simulink model "Simulink_Simulation"  (Simulink 10.1)
settings: Solver=ode23tb  StartTime=0.0  StopTime=3  RelTol=1e-3  EnableMultiTasking=on
undefined symbols (not defined in the file or in its folder): sigbuilder_block
libraries: powerlib x10, powerlib_meascontrol x1
settings Model: Creator=asus1  LastModifiedBy=x64
settings DataIOCC: LimitDataPoints=on
settings DebuggingCC: UnderspecifiedInitializationDetection=Simplified  MergeDetectMultiDrivingBlocksExec=error  SolverPrmCheckMsg=warning
settings GRTTargetCC: CombineOutputUpdateFcns=on  GRTInterface=off
settings ConfigComp: CovSFcnEnable=off
settings SimscapeCC: SimscapeNormalizeSystem=off

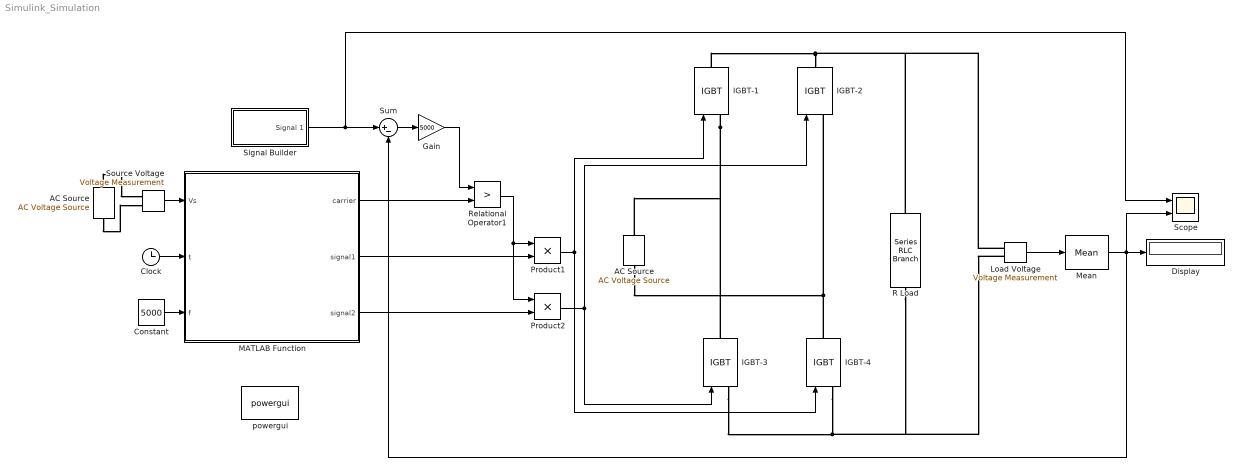
== system Simulink_Simulation ==
  AC Source : powerlib/Electrical Sources/AC Voltage Source  Amplitude=220*sqrt(2)  Phase=0  Frequency=50  SampleTime=0  Measurements=None  BusType=swing  Pref=10e3  Qref=0  Qmin=-inf  Qmax=+inf
  "AC Source " : powerlib/Electrical Sources/AC Voltage Source  Amplitude=220*sqrt(2)  Phase=0  Frequency=50  SampleTime=0  Measurements=None  BusType=swing  Pref=10e3  Qref=0  Qmin=-inf  Qmax=+inf
  "Clock " : Clock
  "Constant " : Constant  Value=5000
  "Display " : Display
  Gain : Gain  Gain=5000
  IGBT-{1..4} (4 alike) : powerlib/Power Electronics/IGBT  Ron=0.001  Lon=0  Vf=0.001  Tf=1e-6  Tt=2e-6  IC=0  Rs=1e5  Cs=inf  Measurements=off
  Load Voltage : powerlib/Measurements/Voltage Measurement  PhasorSimulation=off  OutputType=Complex  PSBequivalent=0
  "MATLAB Function " : MATLAB Function  TreatAsAtomicUnit=on
  Mean : powerlib_meascontrol/Measurements/Mean  Freq=50  Vinit=0  Ts=0
  Product1 : Product
  Product2 : Product
  R Load : powerlib/Elements/Series RLC Branch  LConnTagsString=__new0  RConnTagsString=__new0  BranchType=R  Resistance=10  Inductance=1e-3  SetiL0=off  InitialCurrent=0  Capacitance=1e-6  Setx0=off  InitialVoltage=0  Measurements=None
  Relational Operator1 : RelationalOperator  Operator=>  OutDataTypeStr=boolean  RndMeth=Nearest
  "Scope " : Scope  NumInputPorts=2
  "Signal Builder " : Subsystem  Tag=STV Subsys  LoadFcn=sigbuilder_block('load');  StartFcn=sigbuilder_block('start');  StopFcn=sigbuilder_block('stop');  ClipboardFcn=sigbuilder_block('clipboard');  mask(Sigbuilder block){tuvar=[0:10]}
      mask help: Simulink:masks:SigbuilderBlock_MD
      mask init:
      | if ~strcmp(get_param(bdroot(gcbh),'SimulationStatus'),'stopped') tuvar = sigbuilder_block('maskInit'); end
      settings: CopyFcn=sigbuilder_block('copy');  DeleteFcn=sigbuilder_block('delete');  ModelCloseFcn=sigbuilder_block('modelClose');  PreSaveFcn=sigbuilder_block('preSave');  PauseFcn=sigbuilder_block('pause');  ContinueFcn=sigbuilder_block('continue');  NameChangeFcn=sigbuilder_block('namechange');  OpenFcn=sigbuilder_block('open',[0 30 1152 561.6 ]);  CloseFcn=sigbuilder_block('close');
      mask Display: plot(0, 0, 100, 100,[2, 2, 32, 32, 2], [68, 8, 8, 68, 68],[32, 2], [38, 38], [32, 19, 2],[53, 60, 44], [32, 17, 17, 2],[16, 16, 31, 31]);txt = getActiveGroup(gcbh);text(2, 100, txt,'verticalAlignment', 'top');
  Source Voltage : powerlib/Measurements/Voltage Measurement  PhasorSimulation=off  OutputType=Complex  PSBequivalent=0
  Sum : Sum  Inputs=|+-
  powergui : powerlib/powergui  Priority=1  SimulationMode=Discrete  SampleTime=1e-6  frequency=60  Iterations=50  frequencyindice=50  Pbase=100e6  ErrMax=1e-4  UnitsV=kV  UnitsW=MW  buscounter=0  FunctionMessages=off  echomessages=off  EnableUseOfTLC=off  CurrentSourceSwitches=off  DisableSnubberDevices=off  DisableRonSwitches=off  DisableVfSwitches=off  DisplayEquations=off  AutomaticDiscreteSolvers=off  SolverType=Tustin  Interpol=off  ExternalGateDelay=off  methode=off  Ts=100  x0status=blocks  SPID=off  SwTol=0  HookPort=off  NonlinearTolerance=1e-4  nMaxIteration=100  ContinueOnMaxIteration=off  RestoreLinks=warning  ResistiveCurrentMeasurement=off  Frange=[0:2:500]  Ylog=off  Xlog=on  ShowGrid=off  save=off  variable=ZData  structure=0  ZoomFFT=off  StartTime=0.0  cycles=1  DisplayStyle=1  fundamental=60  FreqAxis=off  MaxFrequency=1000  frequencyindicesteady=1  RmsSteady=1  display=off
  wires:
  Mean/1 -> "Scope "/2, Sum/2, "Display "/1
  Source Voltage/1 -> "MATLAB Function "/1(Vs)
  Load Voltage/1 -> Mean/1
  "Constant "/1 -> "MATLAB Function "/3(f)
  Sum/1 -> Gain/1
  Product2/1 -> IGBT-2/1, IGBT-3/1
  "Clock "/1 -> "MATLAB Function "/2(t)
  Relational Operator1/1 -> Product1/1, Product2/1
  "MATLAB Function "/3(signal2) -> Product2/2
  "MATLAB Function "/2(signal1) -> Product1/2
  "MATLAB Function "/1(carrier) -> Relational Operator1/2
  Gain/1 -> Relational Operator1/1
  Product1/1 -> IGBT-4/1, IGBT-1/1
  "Signal Builder "/1(Signal 1) -> "Scope "/1, Sum/1
  connections:
  IGBT-1/LConn1 -- "AC Source "/RConn1 -- IGBT-3/RConn1
  "AC Source "/LConn1 -- IGBT-2/LConn1 -- IGBT-4/RConn1
  IGBT-3/LConn1 -- R Load/RConn1 -- Load Voltage/LConn2 -- IGBT-4/LConn1
  IGBT-2/RConn1 -- R Load/LConn1 -- Load Voltage/LConn1 -- IGBT-1/RConn1
  AC Source/RConn1 -- Source Voltage/LConn1
  AC Source/LConn1 -- Source Voltage/LConn2

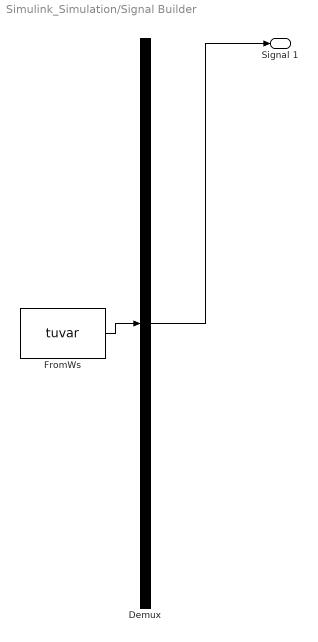
== system Simulink_Simulation/Signal Builder  ==
  Demux : Demux  Tag=STV Demux  Outputs=1
      settings: DisplayOption=none
  FromWs : FromWorkspace  Tag=STV FromWs  VariableName=tuvar  SigBuilderData=DataTag0  VnvData=DataTag1
      SigBuilderData=|
      | common.afterFinalStr = 'Extrapolate'
      | common.sampleTime = 0
      | dataSet.timeRange = [0 10]
      | dataSet.name = 'Group 1'
      | sbobj.Groups.Name = 'Group 1'
      | sbobj.Groups.Signals.Name = 'Signal 1'
      | sbobj.Groups.Signals.XData = [0 0.5 0.5 1 1 1.5 1.5 2 2 2.5 2.5 4 4 6 6 10]
      | sbobj.Groups.Signals.YData = [180 180 140 140 100 100 60 60 20 20 10 10 1 1 0 0]
  Signal 1 : Outport  Tag=STV Outport
  wires:
  Demux/1 -> Signal 1/1
  FromWs/1 -> Demux/1

== matlab function MATLAB Function  ==
  data: Vs input double; carrier output double; t input double; f input double; signal1 output double; signal2 output double
function [carrier, signal1, signal2] = PWM_Generator(Vs, t, f)
% In this program, the triangular wave is in DC signal form within T/2.

% --- Initialization ---
signal1 = 0;
signal2 = 0;

T = 1/f;        % Period
V = 1;          % Amplitude
slope = 2*f*V;  % Slope (m)
carrier = 0;    % Triangular wave (e)

index = fix(t/T); % Cycle index (b)

% --- Triangular Wave Generation ---
% Rising part
if (t >= index*T) && (t <= (index + 0.5)*T)
    carrier = slope * (t - (index + 0.5)*T) + V;
end

% Falling part
if (t > (0.5 + index)*T) && (t <= (index + 1)*T)
    carrier = -slope * (t - (index + 0.5)*T) + V;
end

% Absolute value to make it positive (Unipolar triangle)
carrier = abs(carrier);

% --- PWM Comparator Logic ---
% Compare Control Signal (Vs) with Carrier Wave
if Vs > carrier  % Corrected from '0' to 'carrier' based on Project PDF logic
    signal1 = 1;
    signal2 = 0;
else
    signal1 = 0;
    signal2 = 1;
end
